simulink model "Arrays2"  (Simulink 5.0)
settings: Solver=FixedStepDiscrete  StartTime=0.0  StopTime=10000.0  RelTol=1e-3
settings Model: Creator=scaife  LastModifiedBy=scaife  ExtModeAutoUpdateStatusClock=off

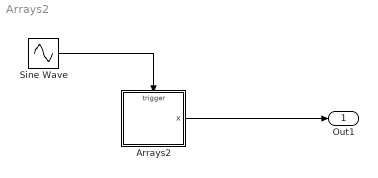
== system Arrays2 ==
  Arrays2 : Stateflow chart
  Sine Wave : Sin  SampleTime=0
  Out1 : Outport
  wires:
  Sine Wave/1 -> Arrays2/Trigger
  Arrays2/1(x) -> Out1/1

== stateflow chart Arrays2 ==
  state A/
    en:x[1][1]++
    x[2][1]--
  state B/
    en:x[1][2]++
    x[2][2]--
  state C/
    en:x[1][3]++
    x[2][3]--
  (default) -> A
  A -> B : E
  B -> C : E
  C -> A : E
  data: x output int32 size=[2 3] [0..100] =1
  events: E input RISING_EDGE_EVENT
